simulink model "SIM_NARENDRA_1_METODO_DIFERENCIAL_RECURSIVO_T2"  (R2015a)
settings: Solver=ode3  StartTime=0.0  StopTime=25  FixedStep=1e-4  RelTol=1e-3
settings Model: Creator=user  LastModifiedBy=user

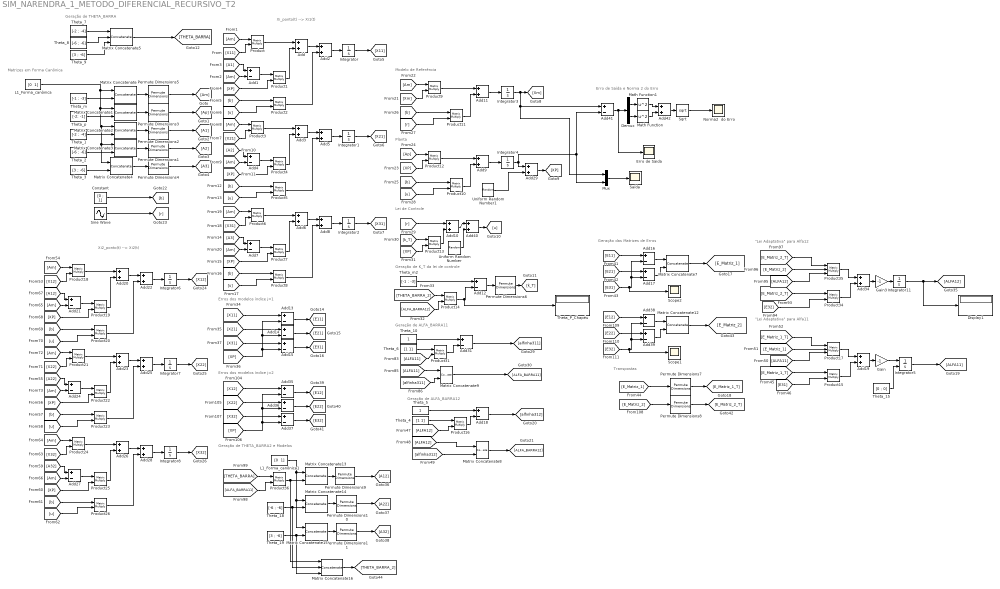
== system SIM_NARENDRA_1_METODO_DIFERENCIAL_RECURSIVO_T2 ==
  note: Erro de Saída e Norma 2 do Erro
  note: Geração de THETA_BARRA
  note: Geração das Matrizes de Erros
  note: "Lei Adaptativa" para Alfa12
  note: "Lei Adaptativa" para Alfa11
  note: Geração de THETA_BARRA2 e Modelos
  note: Erros dos modelos índice j=1
  note: Erros dos modelos índice j=2
  note: Transpostas
  note: Geração de ALFA_BARRA11
  note: Geração de ALFA_BARRA12
  note: Geração de K_T da lei de controle
  note: Lei de Controle
  note: Planta
  note: Modelo de Referência
  note: Matrizes em Forma Canônica
  note: Xi_ponto(t) --> Xi1(t)
  note: Xi2_ponto(t) --> Xi2(t)
  Add{,2..3,5..6,8..11,19..20,22..23,25..26,28..29,34,40,42} (20 alike) : Sum
  Add{1,4,7,12..18,21,24,27,31,35..39,41} (20 alike) : Sum  Inputs=+-
  Constant : Constant  Value=[0 ; 1]
  Demux : Demux  Outputs=2
  Display1 : Display
  Erro de Saida : Scope
      settings: YMin=-0.5  YMax=10.5  SaveName=ScopeData4
  Gain : Gain  Gain=-1
  Gain3 : Gain  Gain=-1
  Integrator : Integrator  InitialCondition=[2 2]
  Integrator1 : Integrator  InitialCondition=[1 0]
  Integrator11 : Integrator
  Integrator2 : Integrator  InitialCondition=[0 0]
  Integrator3 : Integrator
  Integrator4 : Integrator  InitialCondition=[0.01 0.02]
  Integrator5 : Integrator  InitialConditionSource=external
  Integrator6 : Integrator  InitialCondition=[2 2]
  Integrator7 : Integrator  InitialCondition=[1 0]
  Integrator8 : Integrator  InitialCondition=[0 0]
  L1_Forma_canônica : Constant  Value="[0  1]"
  L1_Forma_canônica1 : Constant  Value="[0  1]"
  Math Function : Math  Operator=square  SaturateOnIntegerOverflow=on
  Math Function1 : Math  Operator=square  SaturateOnIntegerOverflow=on
  Matrix Concatenate{,1..4,7,12..15} (10 alike) : Concatenate  Mode=Multidimensional array  ConcatenateDimension=2
  Matrix Concatenate16 : Concatenate  NumInputs=3  Mode=Multidimensional array  ConcatenateDimension=2
  Matrix Concatenate5 : Concatenate  NumInputs=3  Mode=Multidimensional array  ConcatenateDimension=2
  Matrix Concatenate8 : Concatenate
  Matrix Concatenate9 : Concatenate
  Mux : Mux  Inputs=2
  Norma2  do Erro : Scope
      settings: YMin=0.04  YMax=0.063  SaveName=ScopeData3
  Permute Dimensions{1..11} (11 alike) : PermuteDimensions
  Product{,1..16,18..26,31,34,36} (29 alike) : Product  Multiplication=Matrix(*)
  Product17 : Product  Inputs=3  Multiplication=Matrix(*)
  Product35 : Product  Inputs=3  Multiplication=Matrix(*)
  Saída : Scope
      settings: YMin=-0.5  YMax=10.5
  Scope1 : Scope
      settings: YMax=35
  Scope2 : Scope
      settings: YMax=55  SaveName=ScopeData2
  Sine Wave : Sin  Bias=10  Frequency=2  SampleTime=0
  Sqrt : Sqrt  SaturateOnIntegerOverflow=on
  Theta_1 : Constant  Value=[-2 ; -4]
  Theta_10 : Constant
  Theta_15 : Constant  Value=[0 ; 0]  VectorParams1D=off
  Theta_18 : Constant  Value=[-6 ; -6]
  Theta_19 : Constant  Value=[3 ; -6]
  Theta_2 : Constant  Value=[-6 ; -6]
  Theta_3 : Constant  Value=[3 ; -6]
  Theta_4 : Constant  Value=[1 1]  VectorParams1D=off
  Theta_5 : Constant
  Theta_6 : Constant  Value=[1 1]  VectorParams1D=off
  Theta_7 : Constant  Value=[-2 ; -4]
  Theta_8 : Constant  Value=[-6 ; -6]
  Theta_9 : Constant  Value=[3 ; -6]
  Theta_P_Chapéu : Display
  Theta_m : Constant  Value=[-1 ; -3]
  Theta_m2 : Constant  Value=[-1 ; -3]
  Theta_p : Constant  Value=[-2; -1]
  Uniform Random Number : UniformRandomNumber
  Uniform Random Number1 : UniformRandomNumber
  wires:
  Theta_m/1 -> Matrix Concatenate/2
  L1_Forma_canônica/1 -> Matrix Concatenate4/1, Matrix Concatenate3/1, Matrix Concatenate2/1, Matrix Concatenate1/1, Matrix Concatenate/1
  Theta_p/1 -> Matrix Concatenate1/2
  Theta_1/1 -> Matrix Concatenate2/2
  Theta_2/1 -> Matrix Concatenate3/2
  Theta_3/1 -> Matrix Concatenate4/2
  Matrix Concatenate/1 -> Permute Dimensions5/1
  Matrix Concatenate1/1 -> Permute Dimensions3/1
  Matrix Concatenate2/1 -> Permute Dimensions2/1
  Matrix Concatenate3/1 -> Permute Dimensions1/1
  Matrix Concatenate4/1 -> Permute Dimensions4/1
  Permute Dimensions4/1 -> [A3]
  Permute Dimensions1/1 -> [A2]
  Permute Dimensions2/1 -> [A1]
  Permute Dimensions3/1 -> [Ap]
  Permute Dimensions5/1 -> [Am]
  [Am] -> Product/1
  [X11] -> Product/2
  Product/1 -> Add/1
  Product1/1 -> Add/2
  Add1/1 -> Product1/1
  [Am] -> Add1/2
  [A1] -> Add1/1
  [XP] -> Product1/2
  Add/1 -> Add2/1
  Product2/1 -> Add2/2
  [b] -> Product2/1
  [u] -> Product2/2
  Add2/1 -> Integrator/1
  Integrator/1 -> [X11]
  [Am] -> Product3/1
  [X21] -> Product3/2
  Product3/1 -> Add3/1
  Product4/1 -> Add3/2
  Add4/1 -> Product4/1
  [Am] -> Add4/2
  [A2] -> Add4/1
  [XP] -> Product4/2
  Add3/1 -> Add5/1
  Product5/1 -> Add5/2
  [b] -> Product5/1
  [u] -> Product5/2
  Add5/1 -> Integrator1/1
  Integrator1/1 -> [X21]
  [X31] -> Product6/2
  Product6/1 -> Add6/1
  Product7/1 -> Add6/2
  Add7/1 -> Product7/1
  [Am] -> Add7/2
  [A3] -> Add7/1
  [XP] -> Product7/2
  Add6/1 -> Add8/1
  Product8/1 -> Add8/2
  [b] -> Product8/1
  [u] -> Product8/2
  Add8/1 -> Integrator2/1
  Integrator2/1 -> [X31]
  [Am] -> Product6/1
  [Xm] -> Product9/2
  Product9/1 -> Add11/1
  Product11/1 -> Add11/2
  [b] -> Product11/1
  [r] -> Product11/2
  Add11/1 -> Integrator3/1
  [Am] -> Product9/1
  [XP] -> Product12/2
  Product12/1 -> Add9/1
  Product10/1 -> Add9/2
  [b] -> Product10/1
  [u] -> Product10/2
  Add9/1 -> Integrator4/1
  [Ap] -> Product12/1
  [k_T] -> Product13/1
  [XP] -> Product13/2
  Product13/1 -> Add10/2
  [r] -> Add10/1
  Permute Dimensions6/1 -> [k_T]
  [THETA_BARRA_2] -> Product14/1
  [ALFA_BARRA12] -> Product14/2
  Theta_m2/1 -> Add12/1
  Product14/1 -> Theta_P_Chapéu/1, Add12/2
  Add12/1 -> Permute Dimensions6/1
  Theta_7/1 -> Matrix Concatenate5/1
  Theta_8/1 -> Matrix Concatenate5/2
  Theta_9/1 -> Matrix Concatenate5/3
  Matrix Concatenate5/1 -> [THETA_BARRA]
  [X11] -> Add13/1
  [XP] -> Add15/2, Add14/2, Add13/2
  [X21] -> Add14/1
  [X31] -> Add15/1
  Add13/1 -> [E11]
  Add14/1 -> [E21]
  Add15/1 -> [E31]
  [E31] -> Scope2/1, Add17/2, Add16/2
  [E11] -> Add16/1
  [E21] -> Add17/1
  Add17/1 -> Matrix Concatenate7/2
  Add16/1 -> Matrix Concatenate7/1
  [E_Matriz_1] -> Permute Dimensions7/1
  [E_Matriz_1_T] -> Product15/1
  Theta_5/1 -> Add18/1
  Product16/1 -> Add18/2
  [ALFA12] -> Matrix Concatenate8/1
  [alfinha312] -> Matrix Concatenate8/2
  Matrix Concatenate8/1 -> [ALFA_BARRA12]
  Constant/1 -> [b]
  Sine Wave/1 -> [r]
  Matrix Concatenate7/1 -> [E_Matriz_1]
  Mux/1 -> Saída/1
  Product15/1 -> Add19/2
  Add18/1 -> [alfinha312]
  [E31] -> Product15/2
  Permute Dimensions7/1 -> [E_Matriz_1_T]
  [ALFA11] -> Product17/3
  Product17/1 -> Add19/1
  Add19/1 -> Gain/1
  Gain/1 -> Integrator5/1
  [E_Matriz_1] -> Product17/2
  [E_Matriz_1_T] -> Product17/1
  [Am] -> Product18/1
  [X12] -> Product18/2
  Product18/1 -> Add20/1
  Product19/1 -> Add20/2
  Add21/1 -> Product19/1
  [Am] -> Add21/2
  [A12] -> Add21/1
  [XP] -> Product19/2
  Add20/1 -> Add22/1
  Product20/1 -> Add22/2
  [b] -> Product20/1
  [u] -> Product20/2
  Add22/1 -> Integrator6/1
  Integrator6/1 -> [X12]
  [Am] -> Product21/1
  [X22] -> Product21/2
  Product21/1 -> Add23/1
  Product22/1 -> Add23/2
  Add24/1 -> Product22/1
  [Am] -> Add24/2
  [A22] -> Add24/1
  [XP] -> Product22/2
  Add23/1 -> Add25/1
  Product23/1 -> Add25/2
  [b] -> Product23/1
  [u] -> Product23/2
  Add25/1 -> Integrator7/1
  Integrator7/1 -> [X22]
  [X32] -> Product24/2
  Product24/1 -> Add26/1
  Product25/1 -> Add26/2
  Add27/1 -> Product25/1
  [Am] -> Add27/2
  [A32] -> Add27/1
  [XP] -> Product25/2
  Add26/1 -> Add28/1
  Product26/1 -> Add28/2
  [b] -> Product26/1
  [u] -> Product26/2
  Add28/1 -> Integrator8/1
  Integrator8/1 -> [X32]
  [Am] -> Product24/1
  Theta_10/1 -> Add31/1
  Product31/1 -> Add31/2
  [ALFA11] -> Matrix Concatenate9/1
  [alfinha311] -> Matrix Concatenate9/2
  Matrix Concatenate9/1 -> [ALFA_BARRA11]
  [E_Matriz_2_T] -> Product34/1
  Product34/1 -> Add34/2
  [E32] -> Product34/2
  [ALFA12] -> Product35/3
  Product35/1 -> Add34/1
  Add34/1 -> Gain3/1
  Integrator11/1 -> Display1/1, [ALFA12]
  Gain3/1 -> Integrator11/1
  [E_Matriz_2] -> Product35/2
  [E_Matriz_2_T] -> Product35/1
  [THETA_BARRA] -> Product36/1
  [ALFA_BARRA11] -> Product36/2
  [X12] -> Add35/1
  [XP] -> Add35/2, Add36/2, Add37/2
  [X22] -> Add36/1
  [X32] -> Add37/1
  Add35/1 -> [E12]
  Add36/1 -> [E22]
  Add37/1 -> [E32]
  [E_Matriz_2] -> Permute Dimensions8/1
  Permute Dimensions8/1 -> [E_Matriz_2_T]
  [E32] -> Add38/2, Add39/2, Scope1/1
  [E12] -> Add38/1
  [E22] -> Add39/1
  Add39/1 -> Matrix Concatenate12/2
  Add38/1 -> Matrix Concatenate12/1
  Matrix Concatenate12/1 -> [E_Matriz_2]
  Matrix Concatenate15/1 -> Permute Dimensions11/1
  Matrix Concatenate13/1 -> Permute Dimensions9/1
  Product36/1 -> Matrix Concatenate16/1, Matrix Concatenate13/2
  Theta_18/1 -> Matrix Concatenate16/2, Matrix Concatenate14/2
  Theta_19/1 -> Matrix Concatenate16/3, Matrix Concatenate15/2
  L1_Forma_canônica1/1 -> Matrix Concatenate15/1, Matrix Concatenate14/1, Matrix Concatenate13/1
  Matrix Concatenate16/1 -> [THETA_BARRA_2]
  Integrator5/1 -> [ALFA11]
  Add31/1 -> [alfinha311]
  Theta_15/1 -> Integrator5/2
  Theta_6/1 -> Product31/1
  [ALFA11] -> Product31/2
  Theta_4/1 -> Product16/1
  [ALFA12] -> Product16/2
  Add40/1 -> [u]
  Add10/1 -> Add40/1
  Uniform Random Number/1 -> Add40/2
  Matrix Concatenate14/1 -> Permute Dimensions10/1
  Permute Dimensions9/1 -> [A12]
  Permute Dimensions10/1 -> [A22]
  Permute Dimensions11/1 -> [A32]
  Integrator4/1 -> Add41/2, Mux/2, Add29/1
  Integrator3/1 -> Mux/1, Add41/1, [Xm]
  Sqrt/1 -> Norma2  do Erro/1
  Add41/1 -> Erro de Saida/1, Demux/1
  Demux/2 -> Math Function/1
  Demux/1 -> Math Function1/1
  Math Function1/1 -> Add42/1
  Math Function/1 -> Add42/2
  Add42/1 -> Sqrt/1
  Add29/1 -> [XP]
  Uniform Random Number1/1 -> Add29/2
